simulink subsystem "SAC_controller"  (R2025b)
settings: Solver=VariableStepAuto  StartTime=0.0  StopTime=10.0  RelTol=1e-3
undefined symbols (not defined in the file or in its folder): adj, K0, kp, sigma
settings Model: Creator=kawan  LastModifiedBy=kawan

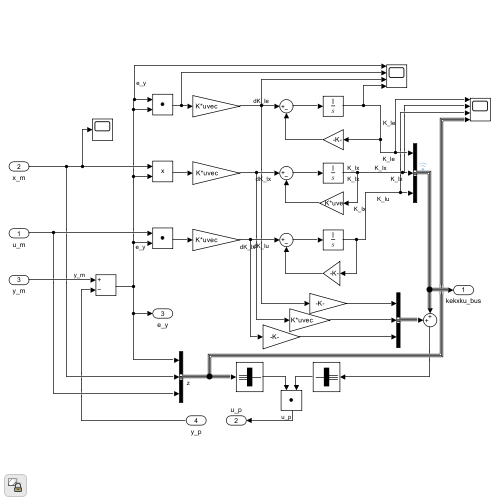
[thumbnail: Simulink's stored preview of the top-level diagram]
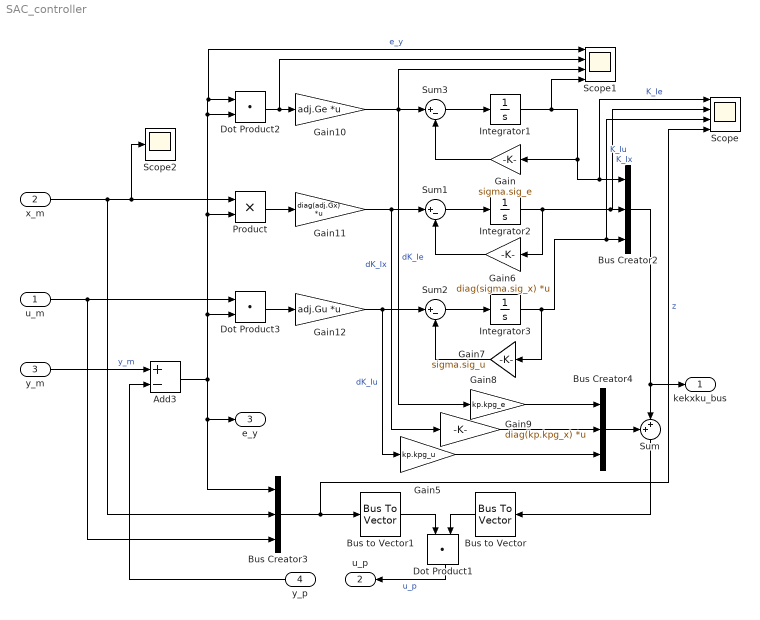
== system SAC_controller ==
  u_m : Inport
  x_m : Inport  Port=2
  y_m : Inport  Port=3
  y_p : Inport  Port=4
  Add3 : Sum  Inputs=+-
  Bus Creator2 : BusCreator  Inputs=3
  Bus Creator3 : BusCreator  Inputs=3
  Bus Creator4 : BusCreator  Inputs=3
  Bus to Vector : BusToVector
  Bus to Vector1 : BusToVector
  Dot Product1 : DotProduct  OutDataTypeStr=Inherit: Inherit via internal rule
  Dot Product2 : DotProduct  OutDataTypeStr=Inherit: Inherit via internal rule
  Dot Product3 : DotProduct  OutDataTypeStr=Inherit: Inherit via internal rule
  Gain : Gain  Gain=sigma.sig_e
  Gain10 : Gain  Gain=adj.Ge  Multiplication=Matrix(K*u) (u vector)
  Gain11 : Gain  Gain=diag(adj.Gx)  Multiplication=Matrix(K*u) (u vector)
  Gain12 : Gain  Gain=adj.Gu  Multiplication=Matrix(K*u) (u vector)
  Gain5 : Gain  Gain=kp.kpg_u
  Gain6 : Gain  Gain=diag(sigma.sig_x)  Multiplication=Matrix(K*u) (u vector)
  Gain7 : Gain  Gain=sigma.sig_u
  Gain8 : Gain  Gain=kp.kpg_e
  Gain9 : Gain  Gain=diag(kp.kpg_x)  Multiplication=Matrix(K*u) (u vector)
  Integrator1 : Integrator  InitialCondition=K0.K0_e
  Integrator2 : Integrator  InitialCondition=K0.K0_x
  Integrator3 : Integrator  InitialCondition=K0.K0_u
  Product : Product
  Scope : Scope  NumInputPorts=4
      settings: ActiveDisplayYMinimum=-0.044735808135574755  ActiveDisplayYMaximum=0.40262227322017285  DataLoggingVariableName=ScopeData7
  Scope1 : Scope  NumInputPorts=4
      settings: ActiveDisplayYMinimum=-0.0083203915598410762  ActiveDisplayYMaximum=0.01565010029101958  DataLoggingVariableName=ScopeData8
  Scope2 : Scope
      settings: ActiveDisplayYMinimum=-4.1899141113705603E-14  ActiveDisplayYMaximum=5.81008588862944E-14  DataLoggingVariableName=ScopeData9
  Sum : Sum  Inputs=++|
  Sum1 : Sum  Inputs=|+-
  Sum2 : Sum  Inputs=|+-
  Sum3 : Sum  Inputs=|+-
  kekxku_bus : Outport
  u_p : Outport  Port=2
  e_y : Outport  Port=3
  wires:
  Gain8/1 -> Bus Creator4/1
  Sum2/1 -> Integrator3/1
  Integrator3/1 -> Gain7/1, Bus Creator2/3, Scope/3  "K_Iu"
  u_m/1 -> Dot Product3/1, Bus Creator3/3
  Gain/1 -> Sum3/2
  x_m/1 -> Bus Creator3/2, Product/1, Scope2/1
  Add3/1 -> Product/2, Dot Product2/2, Dot Product2/1, Scope1/1, Dot Product3/2, Bus Creator3/1, e_y/1  "e_y"
  Bus Creator3/1 -> Bus to Vector1/1, Scope/4  "z"
  Bus Creator2/1 -> kekxku_bus/1, Sum/2
  Integrator2/1 -> Gain6/1, Bus Creator2/2, Scope/2  "K_Ix"
  Gain7/1 -> Sum2/2
  Dot Product1/1 -> u_p/1  "u_p"
  Integrator1/1 -> Gain/1, Bus Creator2/1, Scope/1, Scope1/4  "K_Ie"
  Bus Creator4/1 -> Sum/1
  Gain11/1 -> Gain9/1, Sum1/1  "dK_Ix"
  y_p/1 -> Add3/2
  Dot Product2/1 -> Gain10/1, Scope1/2
  Gain10/1 -> Gain8/1, Sum3/1, Scope1/3  "dK_Ie"
  Gain6/1 -> Sum1/2
  y_m/1 -> Add3/1  "y_m"
  Bus to Vector1/1 -> Dot Product1/1
  Product/1 -> Gain11/1
  Dot Product3/1 -> Gain12/1
  Gain5/1 -> Bus Creator4/3
  Sum/1 -> Bus to Vector/1
  Bus to Vector/1 -> Dot Product1/2
  Gain9/1 -> Bus Creator4/2
  Sum1/1 -> Integrator2/1
  Gain12/1 -> Gain5/1, Sum2/1  "dK_Iu"
  Sum3/1 -> Integrator1/1
